simulink model "position_driver"  (R2015b)
settings: Solver=ode4  StartTime=0.0  StopTime=inf  FixedStep=0.002  RelTol=1e-3
values from neighbouring files (symbols this model uses):
  alpha_pos = 87.7886    [parameters.m]
  Kd_pos = (2*zeta_pos*omega_pos+p_pos-tau_pos)/alpha_pos    (= -0.0467862569855)    [parameters.m]
  Ki_fast = omega_n_fast^2/alpha_fast    (= 0.182256010461)    [parameters.m]
  Ki_pos = (omega_pos^2*p_pos)/alpha_pos    (= 7.29024041846)    [parameters.m]
  Ki_slow = omega_n_slow^2/alpha_slow    (= 0.239027516549)    [parameters.m]
  Kp_fast = (2*zeta_fast*omega_n_fast-tau_fast)/(alpha_fast)    (= -0.502426283139)    [parameters.m]
  Kp_pos = (omega_pos^2+2*zeta_pos*omega_pos*p_pos)/alpha_pos    (= 3.82737621969)    [parameters.m]
  Kp_slow = (2*zeta_slow*omega_n_slow-tau_slow)/(alpha_slow)    (= -0.468023347013)    [parameters.m]
undefined symbols (not defined in the file or in its folder): HIL
libraries: quarc_library x5, simulink x1
settings Model: SimulationMode=external  ExtModeTrigDuration=10000  Creator=flynng  LastModifiedBy=flynng
settings SolverCC: PositivePriorityOrder=on
settings RTWCC: SystemTargetFile=quarc_win64.tlc  TemplateMakefile=quarc_default_tmf  Description=QUARC Win64 Target
settings STFCustomTargetCC: TargetPreCompLibLocation=C:\ProgramData\QUARC\lib\2015b\win64\release  GeneratePreprocessorConditionals=Use local settings  CPPClassGenCompliant=off
settings GRTTargetCC: TargetPreCompLibLocation=C:\ProgramData\QUARC\lib\2015b\win64\release  ParMdlRefBuildCompliant=off  CompOptLevelCompliant=off  CombineOutputUpdateFcns=off  MatFileLogging=off  CPPClassGenCompliant=off  GRTInterface=on  UseToolchainInfoCompliant=off  ExtMode=on  ExtModeMexFile=quarc_comm

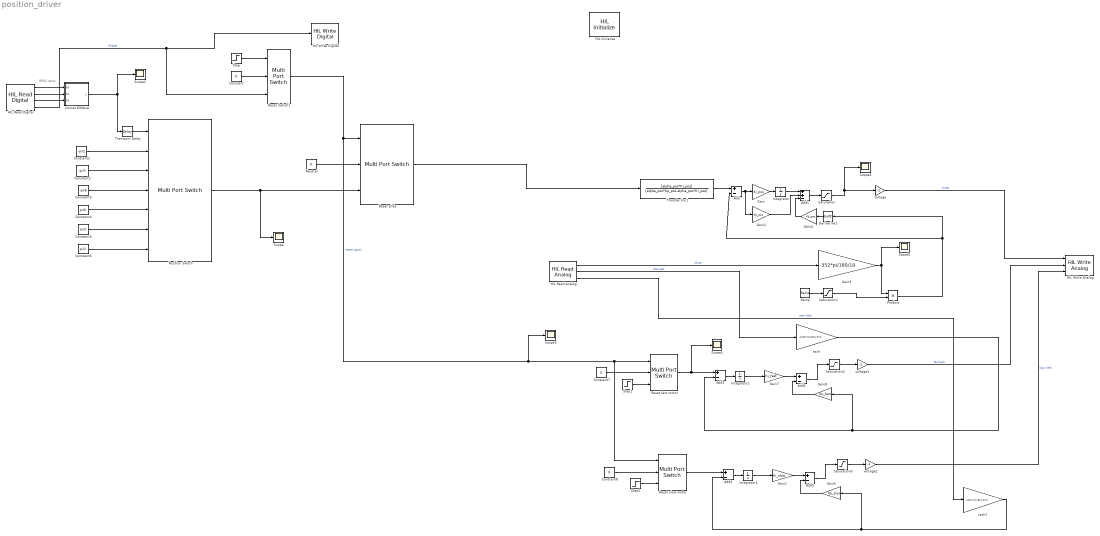
== system position_driver ==
  note: GPIO input
  Add{,2..5} (5 alike) : Sum  Inputs=+-
  Add1 : Sum  Inputs=++-
  Concat BitWise : MATLAB Function  TreatAsAtomicUnit=on
  Constant : Constant  Value=0
  Constant1 : Constant  Value=-pi/2
  Constant2 : Constant  Value=-pi/3
  Constant3 : Constant  Value=-pi/6
  Constant4 : Constant  Value=pi/6
  Constant5 : Constant  Value=pi/3
  Constant6 : Constant  Value=pi/2
  Constant7 : Constant  Value=0
  Constant8 : Constant  Value=0
  Derivative1 : Derivative
  Gain : Gain  Gain=Ki_pos
  Gain1 : Gain  Gain=Ki_slow
  Gain2 : Gain  Gain=Kp_pos
  Gain3 : Gain  Gain=-352*pi/180/10
  Gain4 : Gain  Gain=Kd_pos
  Gain5 : Gain  Gain=Kp_slow
  Gain7 : Gain  Gain=Ki_fast
  Gain8 : Gain  Gain=Kp_fast
  HIL Initialize : quarc_library/Data Acquisition/Generic/Configuration/HIL Initialize  Priority=-99  object_name=HIL-1  board_type=q8_usb  board_number=0  board_options=update_rate=normal;decimation=1  exclusive=off  active=off  hardware_clocks=[0:2]  clock_modes=[]  initial_clock_frequencies=[]  set_clock_params_at_start=off  set_clock_params_at_switch_in=off  set_clock_frequencies_at_start=off  set_clock_frequencies_at_switch_in=off  analog_input_channels=[0:7]  analog_input_maximums=10  analog_input_minimums=-10  set_analog_input_params_at_start=on  set_analog_input_params_at_switch_in=off  analog_output_channels=[0:7]  analog_output_maximums=10  analog_output_minimums=-10  initial_analog_outputs=[0]  final_analog_outputs=[0]  watchdog_analog_outputs=0  set_analog_output_params_at_start=on  set_analog_output_params_at_switch_in=off  set_analog_outputs_at_start=on  set_analog_outputs_at_switch_in=off  set_analog_outputs_at_terminate=on  set_analog_outputs_at_switch_out=off  set_analog_outputs_on_watchdog=off  digital_input_channels=[]  digital_output_channels=[]  digital_output_configuration=[]  initial_digital_outputs=[1]  final_digital_outputs=[1]  watchdog_digital_outputs=[1]  set_digital_output_params_at_start=off  set_digital_output_params_at_switch_in=off  set_digital_outputs_at_start=on  set_digital_outputs_at_switch_in=off  set_digital_outputs_at_terminate=on  set_digital_outputs_at_switch_out=off  set_digital_outputs_on_watchdog=off  encoder_channels=[0:7]  quadrature=[4]  encoder_filter_frequency=[]  initial_encoder_counts=[0]  set_encoder_params_at_start=on  set_encoder_params_at_switch_in=off  set_encoder_counts_at_start=on  set_encoder_counts_at_switch_in=off  pwm_channels=[0:7]  pwm_modes=0  pwm_frequency=99.532799999999995e6/4095  pwm_configuration=[0]  pwm_alignment=[0]  pwm_polarity=[1]  pwm_leading_deadband=[0]  pwm_trailing_deadband=[0]  initial_pwm_outputs=[0]  final_pwm_outputs=[0]  watchdog_pwm_outputs=[0]  set_pwm_params_at_start=on  set_pwm_params_at_switch_in=off  set_pwm_outputs_at_start=on  set_pwm_outputs_at_switch_in=off  set_pwm_outputs_at_terminate=on  set_pwm_outputs_at_switch_out=off  set_pwm_outputs_on_watchdog=off  other_output_channels=[]  initial_other_outputs=[]  final_other_outputs=[]  watchdog_other_outputs=[]  set_other_outputs_at_start=off  set_other_outputs_at_switch_in=off  set_other_outputs_at_terminate=off  set_other_outputs_at_switch_out=off  set_other_outputs_on_watchdog=off
  HIL Read Analog : quarc_library/Data Acquisition/Generic/Immediate I//O/HIL Read Analog  object_name=HIL-1  channels=[0:2]  sample_time=qc_get_step_size  active=on  vector_output=off
  HIL Read Digital : quarc_library/Data Acquisition/Generic/Immediate I//O/HIL Read Digital  object_name=HIL-1  channels=[0:3]  sample_time=qc_get_step_size  active=on  vector_output=off  data_type_mode=Inherit via back propagation  data_type=boolean
      settings: AttributesFormatString=(%<object_name>)
  HIL Write Analog : quarc_library/Data Acquisition/Generic/Immediate I//O/HIL Write Analog  object_name=HIL-1  channels=[0:2]  sample_time=-1  active=off  vector_input=off
  HIL Write Digital : quarc_library/Data Acquisition/Generic/Immediate I//O/HIL Write Digital  object_name=HIL-1  channels=0  sample_time=-1  active=off  vector_input=off
  Integrator : Integrator
  Integrator1 : Integrator
  Integrator2 : Integrator
  Neutral : Constant  Value=0
  Position Switch : MultiPortSwitch  DataPortOrder=Zero-based contiguous  Inputs=6  DiagnosticForDefault=None
  Product : Product
  Ramp : simulink/Sources/Ramp  slope=1  start=0  X0=0
  Reset Switch1 : MultiPortSwitch  DataPortOrder=Zero-based contiguous  Inputs=2
  Reset fast motor : MultiPortSwitch  DataPortOrder=Zero-based contiguous  Inputs=2
  Reset slide : MultiPortSwitch  DataPortOrder=Zero-based contiguous  Inputs=2
  Reset slow motor : MultiPortSwitch  DataPortOrder=Zero-based contiguous  Inputs=2
  Saturation : Saturate  UpperLimit=10  LowerLimit=-10
  Saturation1 : Saturate  UpperLimit=1  LowerLimit=0
  Saturation2 : Saturate  UpperLimit=10  LowerLimit=-10
  Saturation3 : Saturate  UpperLimit=10  LowerLimit=-10
  Scope{,1..5} (6 alike) : Scope
  Step : Step  Time=2  SampleTime=0
  Step1 : Step  Time=0  After=5  SampleTime=0
  Step2 : Step  Time=0  After=5  SampleTime=0
  Transfer Fcn1 : TransferFcn  Numerator=[alpha_pos*Ki_pos]  Denominator=[alpha_pos*Kp_pos alpha_pos*Ki_pos]
  Transport Delay : TransportDelay  DelayTime=2  FixedBuffer=on
  tach : Gain  Gain=-1000*2*pi/60/1.5/70
  tach1 : Gain  Gain=-1000*2*pi/60/1.5/70
  voltage : Gain  Gain=-1
  voltage1 : Gain  Gain=-1
  voltage2 : Gain  Gain=-1
  wires:
  Constant1/1 -> Position Switch/2
  Constant2/1 -> Position Switch/3
  Constant3/1 -> Position Switch/4
  Constant4/1 -> Position Switch/5
  Constant5/1 -> Position Switch/6
  Constant6/1 -> Position Switch/7
  Position Switch/1 -> Reset slide/3, Scope/1
  Concat BitWise/1(y) -> Transport Delay/1, Scope2/1
  HIL Read Digital/1 -> Concat BitWise/1(b0)
  HIL Read Digital/2 -> Concat BitWise/2(b1)
  HIL Read Digital/3 -> Concat BitWise/3(b2)
  Add1/1 -> Saturation/1
  Derivative1/1 -> Gain4/1
  Gain4/1 -> Add1/3
  Add/1 -> Gain2/1, Gain/1
  Gain/1 -> Integrator/1
  Gain2/1 -> Add1/2
  Integrator/1 -> Add1/1
  Transfer Fcn1/1 -> Add/1
  Saturation/1 -> Scope4/1, voltage/1
  voltage/1 -> HIL Write Analog/1  "chute"
  HIL Read Analog/1 -> Gain3/1  "chute"
  Reset slide/1 -> Transfer Fcn1/1
  Gain3/1 -> Product/1, Scope5/1
  HIL Read Digital/4 -> Reset Switch1/3, HIL Write Digital/1  "!Reset"
  Step/1 -> Reset Switch1/1
  Constant/1 -> Reset Switch1/2
  Reset Switch1/1 -> Scope3/1, Reset slow motor/1, Reset fast motor/1, Reset slide/1  "!reset signal"
  Neutral/1 -> Reset slide/2
  Ramp/1 -> Saturation1/1
  Saturation1/1 -> Product/2
  Product/1 -> Add/2, Derivative1/1
  Transport Delay/1 -> Position Switch/1
  tach/1 -> Gain8/1, Add3/2
  Add3/1 -> Integrator2/1
  Integrator2/1 -> Gain7/1
  Gain7/1 -> Add4/1
  Add4/1 -> Saturation2/1
  Gain8/1 -> Add4/2
  Saturation2/1 -> voltage1/1
  voltage1/1 -> HIL Write Analog/2  "fast belt"
  HIL Read Analog/2 -> tach/1  "fast belt"
  Step1/1 -> Reset fast motor/3
  Reset fast motor/1 -> Scope1/1, Add3/1
  Constant7/1 -> Reset fast motor/2
  tach1/1 -> Gain5/1, Add2/2
  Add2/1 -> Integrator1/1
  Integrator1/1 -> Gain1/1
  Gain1/1 -> Add5/1
  Add5/1 -> Saturation3/1
  Gain5/1 -> Add5/2
  Saturation3/1 -> voltage2/1
  voltage2/1 -> HIL Write Analog/3  "slow belt"
  HIL Read Analog/3 -> tach1/1  "slow belt"
  Step2/1 -> Reset slow motor/3
  Reset slow motor/1 -> Add2/1
  Constant8/1 -> Reset slow motor/2

== matlab function position_driver/Concat BitWise ==
  data: b0 input; y output; b1 input; b2 input
function y = fcn(b0, b1, b2)
%#codegen

y = b0 + b1 * 2 + b2 * 4; 
% since apparently we don't have a licence to shift bits.
